simulink model "G6A_Einstiegsaufgabe_Informationstechnik1"  (R2018b)
settings: Solver=FixedStepDiscrete  StartTime=0.0  StopTime=10.0  RelTol=1e-3  EnableMultiTasking=on
libraries: commutil2 x12, c280xlib x3, c2833xlib x2, powerlib_extras x2, c2000lib x1
settings Model: ExtModeTrigDuration=8  Creator=maxth  LastModifiedBy=maxth
settings SolverCC: AutoInsertRateTranBlk=on
settings DataIOCC: LimitDataPoints=on  SaveFormat=Array  SaveOutput=off  SaveTime=off
settings OptimizationCC: DefaultUnderspecifiedDataType=single  ExpressionDepthLimit=2147483647  LifeSpan=1  MaxStackSize=512
settings DebuggingCC: UnderspecifiedInitializationDetection=Classic  MergeDetectMultiDrivingBlocksExec=none  SolverPrmCheckMsg=warning  StateNameClashWarn=warning  SFUnexpectedBacktrackingDiag=warning  SFNoUnconditionalDefaultTransitionDiag=warning  SFExecutionAtInitializationDiag=none
settings HardwareCC: ProdBitPerChar=16  ProdBitPerInt=16  ProdBitPerPointer=32  ProdBitPerSizeT=32  ProdBitPerPtrDiffT=32  ProdLargestAtomicInteger=Integer  ProdLargestAtomicFloat=None  ProdWordSize=16  ProdLongLongMode=on  ProdHWDeviceType=Texas Instruments->C2000  TargetBitPerChar=16  TargetBitPerInt=16  TargetLargestAtomicInteger=Integer  TargetIntDivRoundTo=Zero  TargetEndianess=LittleEndian  TargetWordSize=16  TargetHWDeviceType=Texas Instruments->C2000  ProdEqTarget=off
settings ModelReferenceCC: PropagateSignalLabelsOutOfModel=off
settings SFSimCC: SimCustomSourceCode="#include \"i2c_reset.c\""  SimCustomHeaderCode="#include \"i2c_reset.h\""  SimUseLocalCustomCode=off  MATLABDynamicMemAlloc=off
settings RTWCC: SystemTargetFile=ert.tlc  HardwareBoard=TI Delfino F2833x  TemplateMakefile=ert_default_tmf  RTWUseLocalCustomCode=off  RTWUseSimCustomCode=on  CustomSourceCode="#include \"i2c_reset.c\""  CustomHeaderCode="#include \"i2c_reset.h\""  Toolchain=Texas Instruments Code Composer Studio (C2000)
settings CodeAppCC: IgnoreCustomStorageClasses=off  CustomSymbolStrType=$N$R$M  StateflowObjectComments=on  InternalIdentifier=Classic
settings ERTTargetCC: CodeReplacementLibrary=TI C28x  MultiwordLength=2048  ParMdlRefBuildCompliant=off  CPPClassGenCompliant=off  ConvertIfToSwitch=off  SuppressUnreachableDefaultCases=off
settings ConfigComp: CovMetricSettings=dw  CovHtmlReporting=on  CovSaveCumulativeToWorkspaceVar=on  CovSaveSingleToWorkspaceVar=on  CovExternalEMLEnable=off

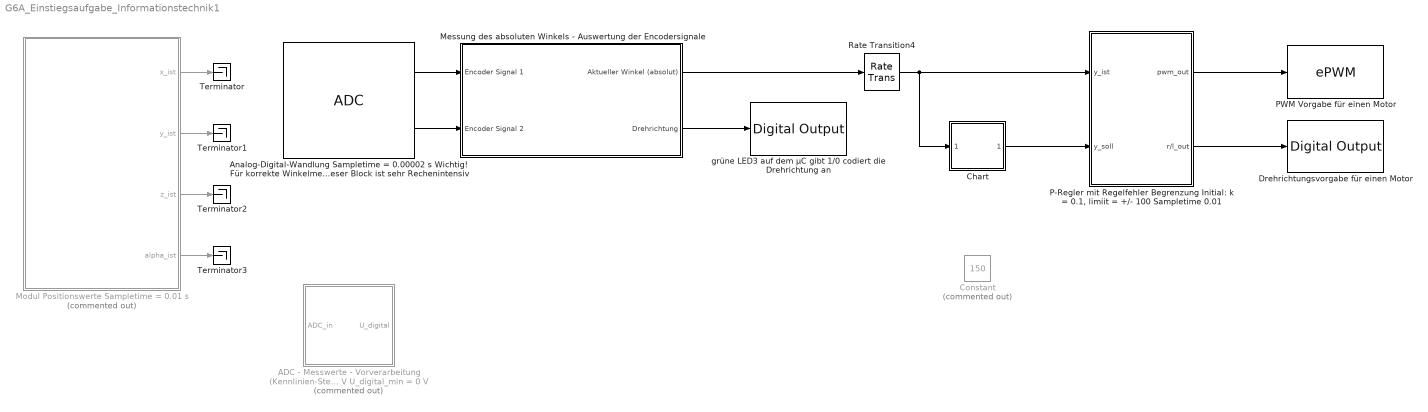
== system G6A_Einstiegsaufgabe_Informationstechnik1 ==
  ADC - Messwerte - Vorverarbeitung (Kennlinien-Steigung und Offset-Kompensation) U_digital = (ADC_in - Offset) * 3.546 V / 4096 mit U_digital_max = 3.546 V U_digital_min = 0 V : Subsystem  Commented=on
  "Analog-Digital-Wandlung Sampletime = 0.00002 s Wichtig! Für korrekte Winkelmessung nicht die Sampletime vergrößern Weitere Ports können hinzugefügt werden (Farbsensor, Sharp-Sensoren) Wichtig! Dieser Block ist sehr Rechenintensiv" : c280xlib/ADC  useModule=A  useMode=Sequential  sourceSOC=Software  sourceSOC1=Software  sourceSOC2=ePWMxB  xint2_ADCSOC=31  Ts=0.00002  dType=double  postInterrupt=off  numConversionsSingle=2  numConversionsDouble=1  conv0=ADCINA0  conv1=ADCINA1  conv2=ADCINA2  conv3=ADCINA3  conv4=ADCINA4  conv5=ADCINA5  conv6=ADCINA6  conv7=ADCINA7  conv8=ADCINB0  conv9=ADCINB1  conv10=ADCINB2  conv11=ADCINB3  conv12=ADCINB4  conv13=ADCINB5  conv14=ADCINB6  conv15=ADCINB7  convAB0=ADCINA0 and ADCINB0  convAB1=ADCINA1 and ADCINB1  convAB2=ADCINA2 and ADCINB2  convAB3=ADCINA3 and ADCINB3  convAB4=ADCINA4 and ADCINB4  convAB5=ADCINA5 and ADCINB5  convAB6=ADCINA6 and ADCINB6  convAB7=ADCINA7 and ADCINB7  convA0=ADCINA0  convA1=ADCINA1  convA2=ADCINA5  convA3=ADCINA3  convA4=ADCINA5  convA5=ADCINA5  convA6=ADCINA6  convA7=ADCINA7  convB0=ADCINB0  convB1=ADCINB1  convB2=ADCINB2  convB3=ADCINB3  convB4=ADCINB4  convB5=ADCINB5  convB6=ADCINB6  convB7=ADCINB7  c28xmultiPort=on  endma=off  chdma=1
      settings: SourceProductName=Embedded Coder Support Package for Texas Instruments C2000 Processors  SourceProductBaseCode=TIC2000
  Chart : Stateflow chart  TreatAsAtomicUnit=on
  Constant : Constant  Commented=on  Value=150
  Drehrichtungsvorgabe für einen Motor : c2833xlib/Digital Output  GPIO_Number=GPIO16~GPIO23  GPIO_Bit0=off  GPIO_BIT0_Toggle=off  GPIO_Bit1=off  GPIO_BIT1_Toggle=off  GPIO_Bit2=off  GPIO_BIT2_Toggle=off  GPIO_Bit3=off  GPIO_BIT3_Toggle=off  GPIO_Bit4=off  GPIO_BIT4_Toggle=off  GPIO_Bit5=on  GPIO_BIT5_Toggle=off  GPIO_Bit6=off  GPIO_BIT6_Toggle=off  GPIO_Bit7=off  GPIO_BIT7_Toggle=off
      settings: SourceProductName=Embedded Coder Support Package for Texas Instruments C2000 Processors  SourceProductBaseCode=TIC2000
  Messung des absoluten Winkels - Auswertung der Encodersignale : Subsystem
  Modul Positionswerte Sampletime = 0.01 s : Subsystem  Commented=on
  "P-Regler mit Regelfehler Begrenzung Initial: k = 0.1, limiit = +/- 100 Sampletime 0.01" : Subsystem
  "PWM Vorgabe für einen Motor " : c280xlib/ePWM  checkMode=off  useModule=ePWM2  periodUnits=Clock cycles  timerSource=Specify via dialog  timerPeriod_clk=64000  timerPeriod_sec=0.0001  tbshadow=Counter equals to zero  countingMode=Up  phaseActiveEnable=Disable  phaseDirection=Count down after sync  phaseActive=0  synchronizationEnable=off  synchronizationOption=Disable  clockPrescale=1  HSclockPrescale=1  ePWMxAStatus=off  CMPAUnits=Clock cycles  CMPASource=Specify via dialog  CMPAValue_per=50  CMPAValue_clk=32000  enCMPAshadow=Counter equals to zero  ePWMxAactionLogic1=Do nothing  ePWMxAactionLogic2=Clear  ePWMxAactionLogic3=Set  ePWMxAactionLogic4=Do nothing  ePWMxAactionLogic5=Do nothing  ePWMxAactionLogic6=Do nothing  ePWMxALoadMode=Load on counter equals to zero (CTR=Zero)  ePWMxACSFenable=off  ePWMxACSFvalue=Forcing disable  ePWMxASFreload=Zero  enHRPWM=off  HRPWM_LoadMode=Counter equals to zero (CTR=ZERO)  HRPWM_CTLMode=Phase control mode  HRPWM_EDGMode=Both edge  enSFO=on  ePWMxBStatus=on  CMPBUnits=Percentages  CMPBSource=Input port  CMPBValue_per=0  CMPBValue_clk=32000  enCMPBshadow=Counter equals to zero  ePWMxBactionLogic1=Do nothing  ePWMxBactionLogic2=Set  ePWMxBactionLogic3=Do nothing  ePWMxBactionLogic4=Do nothing  ePWMxBactionLogic5=Clear  ePWMxBactionLogic6=Do nothing  ePWMxBLoadMode=Load on counter equals to zero (CTR=Zero)  ePWMxBCSFenable=off  ePWMxBCSFvalue=Forcing disable  ePWMxBSFreload=Zero  enableDBePWMxA=off  enableDBePWMxB=off  DBpolarity=Active high (AH)  DBedgeDelay=Positive  DBSource_ePWMxA=ePWMxA  DBSource_ePWMxB=ePWMxA  DBperiodSource=Specify via dialog  REDperiod=0  FEDperiod=0  adcstartModuleA=off  adcrequestEventA=First event  adcstartEventA=Counter equals to zero (CTR=Zero)  adcstartModuleB=off  adcrequestEventB=First event  adcstartEventB=Counter equals to zero (CTR=Zero)  intEn=off  intPrd=First event  intSel=Counter equals to zero (CTR=Zero)  chopperEnable=off  chopperFrequency=1  chopperFirstwidth=1  chopperDuty=12.5%  tripZonesource=Specify via dialog  tzselOSHT1=off  tzselOSHT2=off  tzselOSHT3=off  tzselOSHT4=off  tzselOSHT5=off  tzselOSHT6=off  tzselCBC1=off  tzselCBC2=off  tzselCBC3=off  tzselCBC4=off  tzselCBC5=off  tzselCBC6=off  enTzOstIntr=off  enTzCbcIntr=off  ePWMxAforced=No action  ePWMxBforced=No action  timerPeriod=-1  ePWMxAValue=0  ePWMxBValue=0  tripZoneoption=One-shot trip (OSHT)
      settings: SourceProductName=Embedded Coder Support Package for Texas Instruments C2000 Processors  SourceProductBaseCode=TIC2000
  Rate Transition4 : RateTransition  OutPortSampleTime=0.01
  Terminator{,1..3} (4 alike) : Terminator
  grüne LED3 auf dem µC gibt 1/0 codiert die Drehrichtung an : c2833xlib/Digital Output  GPIO_Number=GPIO32~GPIO39  GPIO_Bit0=off  GPIO_BIT0_Toggle=off  GPIO_Bit1=off  GPIO_BIT1_Toggle=off  GPIO_Bit2=on  GPIO_BIT2_Toggle=off  GPIO_Bit3=off  GPIO_BIT3_Toggle=off  GPIO_Bit4=off  GPIO_BIT4_Toggle=off  GPIO_Bit5=off  GPIO_BIT5_Toggle=off  GPIO_Bit6=off  GPIO_BIT6_Toggle=off  GPIO_Bit7=off  GPIO_BIT7_Toggle=off
      settings: SourceProductName=Embedded Coder Support Package for Texas Instruments C2000 Processors  SourceProductBaseCode=TIC2000
  wires:
  "Analog-Digital-Wandlung Sampletime = 0.00002 s Wichtig! Für korrekte Winkelmessung nicht die Sampletime vergrößern Weitere Ports können hinzugefügt werden (Farbsensor, Sharp-Sensoren) Wichtig! Dieser Block ist sehr Rechenintensiv"/2 -> Messung des absoluten Winkels - Auswertung der Encodersignale/2(Encoder Signal 2)
  "P-Regler mit Regelfehler Begrenzung Initial: k = 0.1, limiit = +/- 100 Sampletime 0.01"/2(r/l_out) -> Drehrichtungsvorgabe für einen Motor/1
  Messung des absoluten Winkels - Auswertung der Encodersignale/1(Aktueller Winkel (absolut)) -> Rate Transition4/1
  "Analog-Digital-Wandlung Sampletime = 0.00002 s Wichtig! Für korrekte Winkelmessung nicht die Sampletime vergrößern Weitere Ports können hinzugefügt werden (Farbsensor, Sharp-Sensoren) Wichtig! Dieser Block ist sehr Rechenintensiv"/1 -> Messung des absoluten Winkels - Auswertung der Encodersignale/1(Encoder Signal 1)
  Messung des absoluten Winkels - Auswertung der Encodersignale/2(Drehrichtung) -> grüne LED3 auf dem µC gibt 1/0 codiert die Drehrichtung an/1
  "P-Regler mit Regelfehler Begrenzung Initial: k = 0.1, limiit = +/- 100 Sampletime 0.01"/1(pwm_out) -> "PWM Vorgabe für einen Motor "/1
  Modul Positionswerte Sampletime = 0.01 s/1(x_ist) -> Terminator/1
  Modul Positionswerte Sampletime = 0.01 s/2(y_ist) -> Terminator1/1
  Modul Positionswerte Sampletime = 0.01 s/3(z_ist) -> Terminator2/1
  Modul Positionswerte Sampletime = 0.01 s/4(alpha_ist) -> Terminator3/1
  Rate Transition4/1 -> Chart/1(change), "P-Regler mit Regelfehler Begrenzung Initial: k = 0.1, limiit = +/- 100 Sampletime 0.01"/1(y_ist)
  Chart/1(angle) -> "P-Regler mit Regelfehler Begrenzung Initial: k = 0.1, limiit = +/- 100 Sampletime 0.01"/2(y_soll)

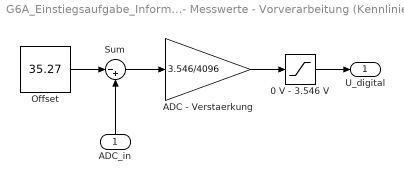
== system G6A_Einstiegsaufgabe_Informationstechnik1/ADC - Messwerte - Vorverarbeitung (Kennlinien-Steigung und Offset-Kompensation) U_digital = (ADC_in - Offset) * 3.546 V // 4096 mit U_digital_max = 3.546 V U_digital_min = 0 V ==
  ADC_in : Inport
  0 V - 3.546 V : Saturate  UpperLimit=3.546  LowerLimit=0
  ADC - Verstaerkung : Gain  Gain=3.546/4096
  Offset : Constant  Value=35.27
  Sum : Sum  Inputs=|-+
  U_digital : Outport
  wires:
  ADC - Verstaerkung/1 -> 0 V - 3.546 V/1
  Sum/1 -> ADC - Verstaerkung/1
  Offset/1 -> Sum/1
  0 V - 3.546 V/1 -> U_digital/1
  ADC_in/1 -> Sum/2

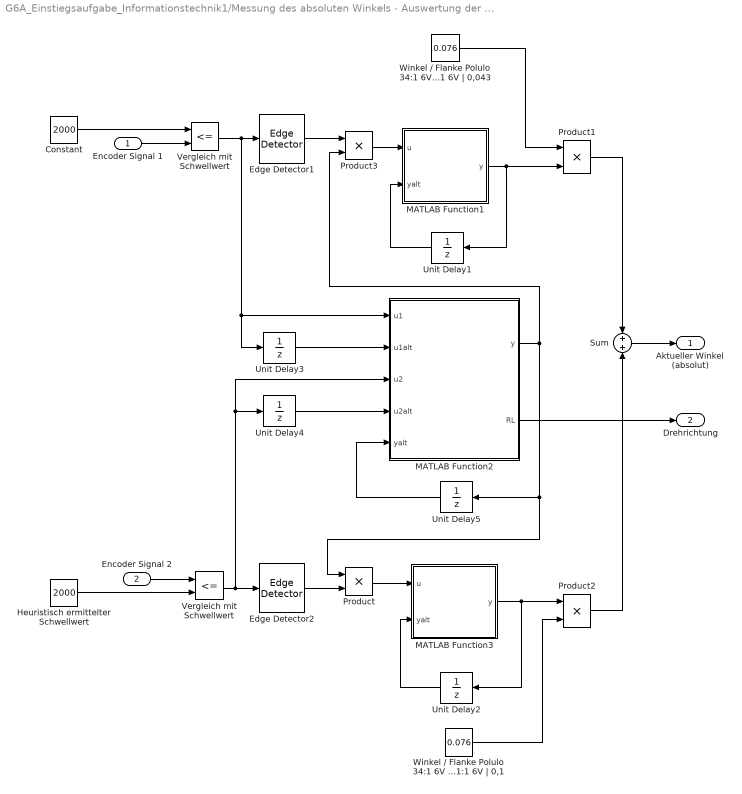
== system G6A_Einstiegsaufgabe_Informationstechnik1/Messung des absoluten Winkels - Auswertung der Encodersignale ==
  Encoder Signal 1 : Inport
  Encoder Signal 2 : Inport  Port=2
  Constant : Constant  Value=2000
  Edge Detector1 : powerlib_extras/Control  Blocks/Edge Detector  model=Either  ic=0
  Edge Detector2 : powerlib_extras/Control  Blocks/Edge Detector  model=Either  ic=0
  Heuristisch ermittelter Schwellwert : Constant  Value=2000
  MATLAB Function1 : MATLAB Function  TreatAsAtomicUnit=on
  MATLAB Function2 : MATLAB Function  TreatAsAtomicUnit=on
  MATLAB Function3 : MATLAB Function  TreatAsAtomicUnit=on
  Product{,1..3} (4 alike) : Product  RndMeth=Zero
  Sum : Sum  Inputs=+|+
  Unit Delay{1..5} (5 alike) : UnitDelay  SampleTime=-1
  Vergleich mit Schwellwert : RelationalOperator  Operator=<=  OutDataTypeStr=boolean  RndMeth=Nearest
  Vergleich mit Schwellwert : RelationalOperator  Operator=<=  OutDataTypeStr=boolean  RndMeth=Nearest
  Winkel / Flanke Polulo 34:1 6V | 0,22 Polulo 74:1 6V | 0,1 Polulo 98:1 6V | 0,076 Polulo 171:1 6V | 0,043 : Constant  Value=0.076
  Winkel / Flanke Polulo 34:1 6V | 0,22 Polulo 74:1 6V | 0,1 Polulo 98:1 6V | 0,076 Polulo 171:1 6V | 0,1 : Constant  Value=0.076
  Aktueller Winkel (absolut) : Outport
  Drehrichtung : Outport  Port=2
  wires:
  Vergleich mit Schwellwert/1 -> Unit Delay4/1, MATLAB Function2/3(u2), Edge Detector2/1
  Sum/1 -> Aktueller Winkel (absolut)/1
  Vergleich mit Schwellwert/1 -> Edge Detector1/1, Unit Delay3/1, MATLAB Function2/1(u1)
  Heuristisch ermittelter Schwellwert/1 -> Vergleich mit Schwellwert/2
  Unit Delay2/1 -> MATLAB Function3/2(yalt)
  Encoder Signal 1/1 -> Vergleich mit Schwellwert/2
  MATLAB Function3/1(y) -> Unit Delay2/1, Product2/1
  Product1/1 -> Sum/1
  Constant/1 -> Vergleich mit Schwellwert/1
  Encoder Signal 2/1 -> Vergleich mit Schwellwert/1
  Product2/1 -> Sum/2
  Unit Delay1/1 -> MATLAB Function1/2(yalt)
  MATLAB Function1/1(y) -> Product1/2, Unit Delay1/1
  Winkel / Flanke Polulo 34:1 6V | 0,22 Polulo 74:1 6V | 0,1 Polulo 98:1 6V | 0,076 Polulo 171:1 6V | 0,043/1 -> Product1/1
  Product3/1 -> MATLAB Function1/1(u)
  Product/1 -> MATLAB Function3/1(u)
  Edge Detector1/1 -> Product3/1
  Unit Delay3/1 -> MATLAB Function2/2(u1alt)
  Unit Delay4/1 -> MATLAB Function2/4(u2alt)
  Edge Detector2/1 -> Product/2
  MATLAB Function2/1(y) -> Product/1, Unit Delay5/1, Product3/2
  Winkel / Flanke Polulo 34:1 6V | 0,22 Polulo 74:1 6V | 0,1 Polulo 98:1 6V | 0,076 Polulo 171:1 6V | 0,1/1 -> Product2/2
  MATLAB Function2/2(RL) -> Drehrichtung/1
  Unit Delay5/1 -> MATLAB Function2/5(yalt)

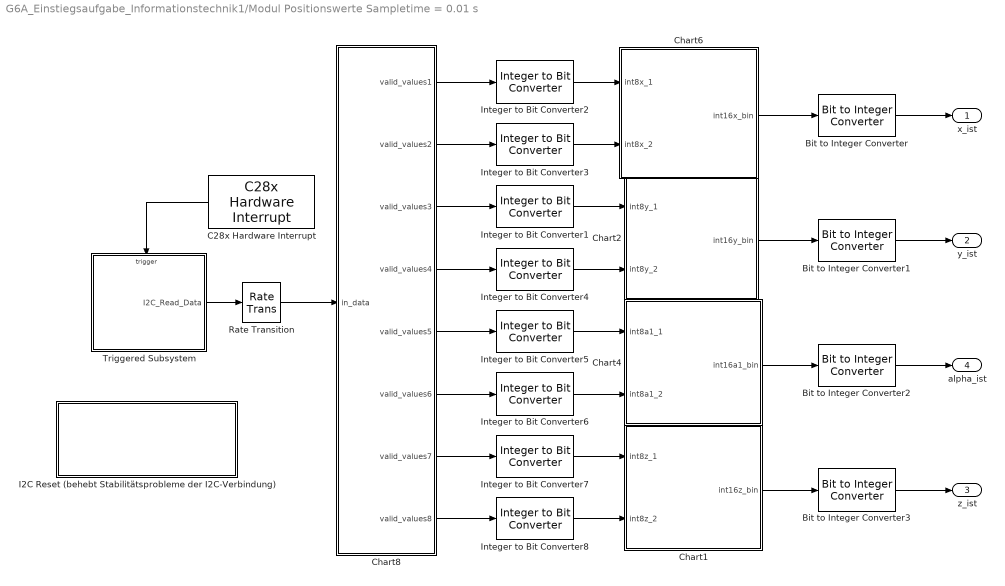
== system G6A_Einstiegsaufgabe_Informationstechnik1/Modul Positionswerte Sampletime = 0.01 s ==
  Bit to Integer Converter{,1..3} (4 alike) : commutil2/Bit to Integer Converter  nbits=16  bitOrder=MSB first  signedOutputValues=Signed  outDtype=Inherit via internal rule  outDtypeSigned=Inherit via internal rule
      settings: SourceProductName=Communications Toolbox
  C28x Hardware Interrupt : c2000lib/Scheduling/C28x Hardware Interrupt  irqnumbers=8  pienumbers=2  irqpriorities=30  irqpreempts=0  showinput=off  dspchiptype=C280X
      settings: SourceProductName=Embedded Coder Support Package for Texas Instruments C2000 Processors  SourceProductBaseCode=TIC2000
  Chart1 : Stateflow chart  TreatAsAtomicUnit=on
  Chart2 : Stateflow chart  TreatAsAtomicUnit=on
  Chart4 : Stateflow chart  TreatAsAtomicUnit=on
  Chart6 : Stateflow chart  TreatAsAtomicUnit=on
  Chart8 : Stateflow chart  TreatAsAtomicUnit=on
  I2C Reset (behebt Stabilitätsprobleme der I2C-Verbindung) : Subsystem
  Integer to Bit Converter{1..8} (8 alike) : commutil2/Integer to Bit Converter  nbits=8  signedInputValues=Unsigned  bitOrder=MSB first  outDtype=uint8
      settings: SourceProductName=Communications Toolbox
  Rate Transition : RateTransition  Deterministic=off  OutPortSampleTime=0.01
  Triggered Subsystem : Subsystem  TreatAsAtomicUnit=on
  x_ist : Outport
  y_ist : Outport  Port=2
  z_ist : Outport  Port=3
  alpha_ist : Outport  Port=4
  wires:
  Integer to Bit Converter7/1 -> Chart1/1(int8z_1)
  Integer to Bit Converter8/1 -> Chart1/2(int8z_2)
  Chart8/7(valid_values7) -> Integer to Bit Converter7/1
  Chart8/8(valid_values8) -> Integer to Bit Converter8/1
  Bit to Integer Converter3/1 -> z_ist/1
  Triggered Subsystem/1(I2C_Read_Data) -> Rate Transition/1
  Chart1/1(int16z_bin) -> Bit to Integer Converter3/1
  Chart4/1(int16a1_bin) -> Bit to Integer Converter2/1
  Chart8/6(valid_values6) -> Integer to Bit Converter6/1
  Bit to Integer Converter2/1 -> alpha_ist/1
  Bit to Integer Converter/1 -> x_ist/1
  Integer to Bit Converter6/1 -> Chart4/2(int8a1_2)
  Integer to Bit Converter5/1 -> Chart4/1(int8a1_1)
  Bit to Integer Converter1/1 -> y_ist/1
  Integer to Bit Converter4/1 -> Chart2/2(int8y_2)
  Integer to Bit Converter2/1 -> Chart6/1(int8x_1)
  Integer to Bit Converter1/1 -> Chart2/1(int8y_1)
  Chart6/1(int16x_bin) -> Bit to Integer Converter/1
  Integer to Bit Converter3/1 -> Chart6/2(int8x_2)
  Chart8/3(valid_values3) -> Integer to Bit Converter1/1
  Chart8/1(valid_values1) -> Integer to Bit Converter2/1
  Chart2/1(int16y_bin) -> Bit to Integer Converter1/1
  Chart8/4(valid_values4) -> Integer to Bit Converter4/1
  Chart8/2(valid_values2) -> Integer to Bit Converter3/1
  Chart8/5(valid_values5) -> Integer to Bit Converter5/1
  C28x Hardware Interrupt/1 -> Triggered Subsystem/Trigger
  Rate Transition/1 -> Chart8/1(in_data)

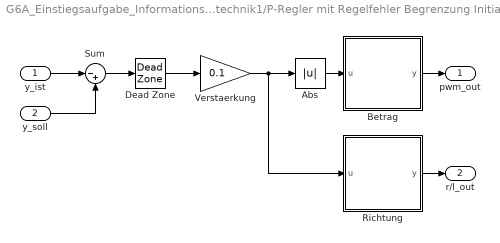
== system G6A_Einstiegsaufgabe_Informationstechnik1/P-Regler mit Regelfehler Begrenzung Initial: k = 0.1, limiit = +//- 100 Sampletime 0.01 ==
  y_ist : Inport
  y_soll : Inport  Port=2
  Abs : Abs  SampleTime=0.01
  Betrag : MATLAB Function  TreatAsAtomicUnit=on  SystemSampleTime=0.01
  Dead Zone : DeadZone  LowerValue=-100  UpperValue=100  SampleTime=0.01  SaturateOnIntegerOverflow=on
  Richtung : MATLAB Function  TreatAsAtomicUnit=on  SystemSampleTime=0.01
  Sum : Sum  Inputs=|-+  SampleTime=0.01
  Verstaerkung : Gain  Gain=0.1  SampleTime=0.01
  pwm_out : Outport
  r/l_out : Outport  Port=2
  wires:
  Betrag/1(y) -> pwm_out/1
  Verstaerkung/1 -> Abs/1, Richtung/1(u)
  Dead Zone/1 -> Verstaerkung/1
  Abs/1 -> Betrag/1(u)
  y_soll/1 -> Sum/2
  Richtung/1(y) -> r/l_out/1
  y_ist/1 -> Sum/1
  Sum/1 -> Dead Zone/1

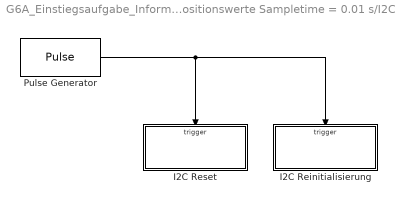
== system G6A_Einstiegsaufgabe_Informationstechnik1/Modul Positionswerte Sampletime = 0.01 s/I2C Reset (behebt Stabilitätsprobleme der I2C-Verbindung) ==
  I2C Reinitialisierung : Subsystem  TreatAsAtomicUnit=on
  I2C Reset : Subsystem  TreatAsAtomicUnit=on
  Pulse Generator : DiscretePulseGenerator  Period=250  SampleTime=0.01
  wires:
  Pulse Generator/1 -> I2C Reset/Trigger, I2C Reinitialisierung/Trigger

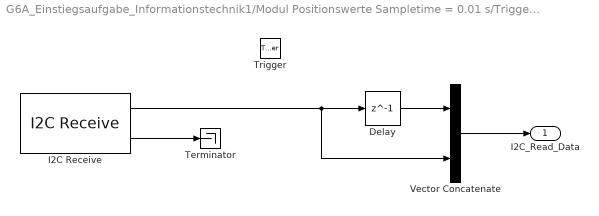
== system G6A_Einstiegsaufgabe_Informationstechnik1/Modul Positionswerte Sampletime = 0.01 s/Triggered Subsystem ==
  Trigger : TriggerPort  TriggerType=function-call  VariantControl=(inherit)
  Delay : Delay  DelayLength=1  InitialCondition=0
  I2C Receive : c280xlib/I2C Receive  selectModule=I2C_A  addrFormat=7-Bit addressing  saSource=Specify via dialog  SAR=80  bitCount=8  dataLength=10  initValue=0  NACK=on  STP=off  STR=on  sampleTime=-1  dataType=uint8
      settings: SourceProductName=Embedded Coder Support Package for Texas Instruments C2000 Processors  SourceProductBaseCode=TIC2000
  Terminator : Terminator
  Vector Concatenate : Concatenate
  I2C_Read_Data : Outport
  wires:
  I2C Receive/2 -> Terminator/1
  I2C Receive/1 -> Vector Concatenate/2, Delay/1
  Delay/1 -> Vector Concatenate/1
  Vector Concatenate/1 -> I2C_Read_Data/1

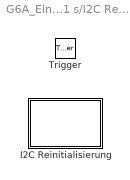
== system G6A_Einstiegsaufgabe_Informationstechnik1/Modul Positionswerte Sampletime = 0.01 s/I2C Reset (behebt Stabilitätsprobleme der I2C-Verbindung)/I2C Reinitialisierung ==
  Trigger : TriggerPort  TriggerType=falling  VariantControl=(inherit)
  I2C Reinitialisierung : MATLAB Function  TreatAsAtomicUnit=on

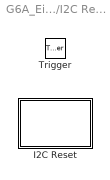
== system G6A_Einstiegsaufgabe_Informationstechnik1/Modul Positionswerte Sampletime = 0.01 s/I2C Reset (behebt Stabilitätsprobleme der I2C-Verbindung)/I2C Reset ==
  Trigger : TriggerPort  VariantControl=(inherit)
  I2C Reset : MATLAB Function  TreatAsAtomicUnit=on

== stateflow chart G6A_Einstiegsaufgabe_Informationstechnik1/Chart ==
  state Start
    angle=0;
  state Winkel1
    angle=30*2/3;
  state Winkel2
    angle=290*2/3;
  (default) -> Start
  Start -> Winkel1 : after(1,sec)
  Winkel2 -> Winkel1 : after(5,sec)[change==angle]
  Winkel1 -> Winkel2 : after(5,sec)[change==angle]
  data: angle output; change input

== matlab function G6A_Einstiegsaufgabe_Informationstechnik1/P-Regler mit Regelfehler Begrenzung Initial: k = 0.1, limiit = +//- 100 Sampletime 0.01/Betrag ==
  settings: updateMethod=DISCRETE  sampleTime=0.01
  data: u input; y output
function y = fcn( u )

if 0.5 < u && u < 60
    y = 60;
elseif u <= 0.5
    y = 0;
elseif u >= 100
    y = 100;
else
    y = abs(u);
end

== matlab function G6A_Einstiegsaufgabe_Informationstechnik1/P-Regler mit Regelfehler Begrenzung Initial: k = 0.1, limiit = +//- 100 Sampletime 0.01/Richtung ==
  settings: updateMethod=DISCRETE  sampleTime=0.01
  data: u input; y output
function y = fcn( u )

if u > 0
    y = 1;
else
    y = 0;
end

== matlab function G6A_Einstiegsaufgabe_Informationstechnik1/Messung des absoluten Winkels - Auswertung der Encodersignale/MATLAB Function1 ==
  data: u input; y output; yalt input
function y = fcn(u, yalt)

y = yalt + u;

== stateflow chart G6A_Einstiegsaufgabe_Informationstechnik1/Modul Positionswerte Sampletime = 0.01 s/Chart1 ==
  state Daten_einlesen
  state x0
  state x1_1
    entry: int16z_bin[0] = int8z_1[0];
    int16z_bin[1] = int8z_1[1];
    int16z_bin[2] = int8z_1[2];
    int16z_bin[3] = int8z_1[3];
    int16z_bin[4] = int8z_1[4];
    int16z_bin[5] = int8z_1[5]
    int16z_bin[6] = int8z_1[6];
    int16z_bin[7] = int8z_1[7];
    int16z_bin[8] = int8z_2[0];
    int16z_bin[9] = int8z_2[1];
    int16z_bin[10] = int8z_2[2];
    int16z_bin[11] = int8z_2[3];
    int16z_bin[12] = int8z_2[4];
    int16z_bin[13] = int8z_2[5]
    int16z_bin[14] = int8z_2[6];
    int16z_bin[15] = int8z_2[7];
  x0 -> Daten_einlesen
  (default) -> x0
  Daten_einlesen -> x1_1
  x1_1 -> Daten_einlesen
  data: int8z_1 input size=8; int8z_2 input size=8; int16z_bin output size=16 =0

== stateflow chart G6A_Einstiegsaufgabe_Informationstechnik1/Modul Positionswerte Sampletime = 0.01 s/Chart2 ==
  state Daten_einlesen
  state x0
  state x1_1
    entry: int16y_bin[0] = int8y_1[0];
    int16y_bin[1] = int8y_1[1];
    int16y_bin[2] = int8y_1[2];
    int16y_bin[3] = int8y_1[3];
    int16y_bin[4] = int8y_1[4];
    int16y_bin[5] = int8y_1[5]
    int16y_bin[6] = int8y_1[6];
    int16y_bin[7] = int8y_1[7];
    int16y_bin[8] = int8y_2[0];
    int16y_bin[9] = int8y_2[1];
    int16y_bin[10] = int8y_2[2];
    int16y_bin[11] = int8y_2[3];
    int16y_bin[12] = int8y_2[4];
    int16y_bin[13] = int8y_2[5]
    int16y_bin[14] = int8y_2[6];
    int16y_bin[15] = int8y_2[7];
  x0 -> Daten_einlesen
  (default) -> x0
  Daten_einlesen -> x1_1
  x1_1 -> Daten_einlesen
  data: int8y_1 input size=8; int8y_2 input size=8; int16y_bin output size=16 =0

== stateflow chart G6A_Einstiegsaufgabe_Informationstechnik1/Modul Positionswerte Sampletime = 0.01 s/Chart4 ==
  state Daten_einlesen
  state x0
  state x1_1
    entry: int16a1_bin[0] = int8a1_1[0];
    int16a1_bin[1] = int8a1_1[1];
    int16a1_bin[2] = int8a1_1[2];
    int16a1_bin[3] = int8a1_1[3];
    int16a1_bin[4] = int8a1_1[4];
    int16a1_bin[5] = int8a1_1[5]
    int16a1_bin[6] = int8a1_1[6];
    int16a1_bin[7] = int8a1_1[7];
    int16a1_bin[8] = int8a1_2[0];
    int16a1_bin[9] = int8a1_2[1];
    int16a1_bin[10] = int8a1_2[2];
    int16a1_bin[11] = int8a1_2[3];
    int16a1_bin[12] = int8a1_2[4];
    int16a1_bin[13] = int8a1_2[5]
    int16a1_bin[14] = int8a1_2[6];
    int16a1_bin[15] = int8a1_2[7];
  x0 -> Daten_einlesen
  (default) -> x0
  Daten_einlesen -> x1_1
  x1_1 -> Daten_einlesen
  data: int8a1_1 input size=8; int8a1_2 input size=8; int16a1_bin output size=16 =0

== matlab function G6A_Einstiegsaufgabe_Informationstechnik1/Messung des absoluten Winkels - Auswertung der Encodersignale/MATLAB Function2 ==
  data: u1 input; u1alt input; u2 input; u2alt input; y output; yalt input double; RL output
function [y, RL] = fcn(u1, u1alt, u2, u2alt, yalt)

y = 1;
RL = 1;

if u1alt == 0 && u2alt == 0 && u1 == 0 && u2 == 0
    y = yalt;
end

if u1alt == 0 && u2alt == 0 && u1 == 0 && u2 == 1
    y = 1;
end

if u1alt == 0 && u2alt == 0 && u1 == 1 && u2 == 0
    y = -1;
end

% if u1alt == 0 && u2alt == 0 && u1 == 1 && u2 == 1
%     y = yalt;   % nicht möglich
% end

if u1alt == 0 && u2alt == 1 && u1 == 0 && u2 == 0
    y = -1;
end

if u1alt == 0 && u2alt == 1 && u1 == 0 && u2 == 1
    y = yalt;
end

% if u1alt == 0 && u2alt == 1 && u1 == 1 && u2 == 0
%     y = yalt;   % nicht möglich
% end

if u1alt == 0 && u2alt == 1 && u1 == 1 && u2 == 1
    y = 1;
end

if u1alt == 1 && u2alt == 0 && u1 == 0 && u2 == 0
    y = 1;
end

% if u1alt == 1 && u2alt == 0 && u1 == 0 && u2 == 1
%     y = yalt;   % nicht möglich
% end

if u1alt == 1 && u2alt == 0 && u1 == 1 && u2 == 0
    y = yalt;
end

if u1alt == 1 && u2alt == 0 && u1 == 1 && u2 == 1
    y = -1;
end

% if u1alt == 1 && u2alt == 1 && u1 == 0 && u2 == 0
%     y = yalt;   % nicht möglich
% end

if u1alt == 1 && u2alt == 1 && u1 == 0 && u2 == 1
    y = -1;
end

if u1alt == 1 && u2alt == 1 && u1 == 1 && u2 == 0
    y = 1;
end

if u1alt == 1 && u2alt == 1 && u1 == 1 && u2 == 1
    y = yalt;
end

if y == 1
    RL = 1;
else
    RL = 0;
end

== stateflow chart G6A_Einstiegsaufgabe_Informationstechnik1/Modul Positionswerte Sampletime = 0.01 s/Chart6 ==
  state Daten_einlesen
  state x0
  state x1_1
    entry: int16x_bin[0] = int8x_1[0];
    int16x_bin[1] = int8x_1[1];
    int16x_bin[2] = int8x_1[2];
    int16x_bin[3] = int8x_1[3];
    int16x_bin[4] = int8x_1[4];
    int16x_bin[5] = int8x_1[5]
    int16x_bin[6] = int8x_1[6];
    int16x_bin[7] = int8x_1[7];
    int16x_bin[8] = int8x_2[0];
    int16x_bin[9] = int8x_2[1];
    int16x_bin[10] = int8x_2[2];
    int16x_bin[11] = int8x_2[3];
    int16x_bin[12] = int8x_2[4];
    int16x_bin[13] = int8x_2[5]
    int16x_bin[14] = int8x_2[6];
    int16x_bin[15] = int8x_2[7];
  x0 -> Daten_einlesen
  (default) -> x0
  Daten_einlesen -> x1_1
  x1_1 -> Daten_einlesen
  data: int8x_1 input size=8; int8x_2 input size=8; int16x_bin output size=16 =0

== stateflow chart G6A_Einstiegsaufgabe_Informationstechnik1/Modul Positionswerte Sampletime = 0.01 s/Chart8 ==
  state wert_erkannt
    entry:
    values_out1[0] = in_data[0];
    values_out1[1] = in_data[1];
    values_out1[2] = in_data[2];
    values_out1[3] = in_data[3];
    values_out1[4] = in_data[4];
    values_out1[5] = in_data[5];
    values_out1[6] = in_data[6];
    values_out1[7] = in_data[7];
    values_out1[8] = in_data[8];
    values_out1[9] = in_data[9];
    values_out1[10] = in_data[10];
    values_out1[11] = in_data[11];
    values_out1[12] = in_data[12];
    values_out1[13] = in_data[13];
    values_out1[14] = in_data[14];
    values_out1[15] = in_data[15];
    values_out1[16] = in_data[16];
    values_out1[17] = in_data[17];
    values_out1[18] = in_data[18];
    values_out1[19] = in_data[19];
  state init
    entry: values_out1[0] = 0;
    values_out1[1] = 0;
    values_out1[2] = 0;
    values_out1[3] = 0;
    values_out1[4] = 0;
    values_out1[5] = 0;
    values_out1[6] = 0;
    values_out1[7] = 0;
    values_out1[8] = 0;
    values_out1[9] = 0;
    values_out1[10] = 0;
    values_out1[11] = 0;
    values_out1[12] = 0;
    values_out1[13] = 0;
    values_out1[14] = 0;
    values_out1[15] = 0;
    values_out1[16] = 0;
    values_out1[17] = 0;
    values_out1[18] = 0;
    values_out1[19] = 0;
  state Anfang_found_Schritt_uebertragen_weglassen_performance
    entry: x_found = x_found +1;
  state x5_valid_data_found1
    entry: valid_values1 = values_out1[search+1];
    valid_values2 = values_out1[search+2];
    valid_values3 = values_out1[search+3];
    valid_values4 = values_out1[search+4];
    valid_values5 = values_out1[search+5];
    valid_values6 = values_out1[search+6];
    valid_values7 = values_out1[search+7];
    valid_values8 = values_out1[search+8];
    zaehler = zaehler +1;
  state wert_erkannt2
    entry:
    search = 0;
    counter = counter + 1;
  state x1_search1
    entry: search = search + 1;
  x5_valid_data_found1 -> wert_erkannt
  (default) -> init
  x1_search1 -> wert_erkannt [order 3]
  init -> wert_erkannt
  Anfang_found_Schritt_uebertragen_weglassen_performance -> x5_valid_data_found1 [order 1] : [((values_out1[search]+values_out1[search+1]+values_out1[search+2]+values_out1[search+3]+values_out1[search+4]+values_out1[search+5]+values_out1[search+6]+values_out1[search+7]+values_out1[search+8])) == values_out1[search+9]]
  Anfang_found_Schritt_uebertragen_weglassen_performance -> x5_valid_data_found1 [order 2] : [((values_out1[search]+values_out1[search+1]+values_out1[search+2]+values_out1[search+3]+values_out1[search+4]+values_out1[search+5]+values_out1[search+6]+values_out1[search+7]+values_out1[search+8])-(256)) == values_out1[search+9]]
  wert_erkannt -> wert_erkannt2
  Anfang_found_Schritt_uebertragen_weglassen_performance -> x5_valid_data_found1 [order 3] : [((values_out1[search]+values_out1[search+1]+values_out1[search+2]+values_out1[search+3]+values_out1[search+4]+values_out1[search+5]+values_out1[search+6]+values_out1[search+7]+values_out1[search+8])-(512)) == values_out1[search+9]]
  Anfang_found_Schritt_uebertragen_weglassen_performance -> x5_valid_data_found1 [order 7] : [((values_out1[search]+values_out1[search+1]+values_out1[search+2]+values_out1[search+3]+values_out1[search+4]+values_out1[search+5]+values_out1[search+6]+values_out1[search+7]+values_out1[search+8])-(768)) == values_out1[search+9]]
  Anfang_found_Schritt_uebertragen_weglassen_performance -> x5_valid_data_found1 [order 6] : [((values_out1[search]+values_out1[search+1]+values_out1[search+2]+values_out1[search+3]+values_out1[search+4]+values_out1[search+5]+values_out1[search+6]+values_out1[search+7]+values_out1[search+8])-(1024)) == values_out1[search+9]]
  Anfang_found_Schritt_uebertragen_weglassen_performance -> x5_valid_data_found1 [order 5] : [((values_out1[search]+values_out1[search+1]+values_out1[search+2]+values_out1[search+3]+values_out1[search+4]+values_out1[search+5]+values_out1[search+6]+values_out1[search+7]+values_out1[search+8])-(1280)) == values_out1[search+9]]
  Anfang_found_Schritt_uebertragen_weglassen_performance -> x5_valid_data_found1 [order 4] : [((values_out1[search]+values_out1[search+1]+values_out1[search+2]+values_out1[search+3]+values_out1[search+4]+values_out1[search+5]+values_out1[search+6]+values_out1[search+7]+values_out1[search+8])-(1536)) == values_out1[search+9]]
  Anfang_found_Schritt_uebertragen_weglassen_performance -> x5_valid_data_found1 [order 8] : [((values_out1[search]+values_out1[search+1]+values_out1[search+2]+values_out1[search+3]+values_out1[search+4]+values_out1[search+5]+values_out1[search+6]+values_out1[search+7]+values_out1[search+8])-(1792)) == values_out1[search+9]]
  Anfang_found_Schritt_uebertragen_weglassen_performance -> x5_valid_data_found1 [order 10] : [((values_out1[search]+values_out1[search+1]+values_out1[search+2]+values_out1[search+3]+values_out1[search+4]+values_out1[search+5]+values_out1[search+6]+values_out1[search+7]+values_out1[search+8])-(2048)) == values_out1[search+9]]
  Anfang_found_Schritt_uebertragen_weglassen_performance -> x1_search1 [order 9]
  wert_erkannt2 -> Anfang_found_Schritt_uebertragen_weglassen_performance [order 1] : [values_out1[search] == 88]
  x1_search1 -> Anfang_found_Schritt_uebertragen_weglassen_performance [order 1] : [values_out1[search] == 88]
  wert_erkannt2 -> x1_search1 [order 2]
  x1_search1 -> x1_search1 [order 2] : [search < 19]
  data: in_data input size=20; values_out1 local int16 size=20; zaehler local int32 =0; search local int16; valid_values1 output int16 size=1; valid_values2 output int16 size=1; valid_values3 output int16 size=1; valid_values4 output int16 size=1; valid_values5 output int16 size=1; valid_values6 output int16 size=1; valid_values7 output int16 size=1; valid_values8 output int16 size=1; counter local int32 =0; x_found local int32 =0

== matlab function G6A_Einstiegsaufgabe_Informationstechnik1/Messung des absoluten Winkels - Auswertung der Encodersignale/MATLAB Function3 ==
  data: u input; y output; yalt input
function y = fcn(u, yalt)

y = yalt + u;

== matlab function G6A_Einstiegsaufgabe_Informationstechnik1/Modul Positionswerte Sampletime = 0.01 s/I2C Reset (behebt Stabilitätsprobleme der I2C-Verbindung)/I2C Reset/I2C Reset ==
function fcn()
%#codegen

coder.ceval( 'reset_i2c' );

== matlab function G6A_Einstiegsaufgabe_Informationstechnik1/Modul Positionswerte Sampletime = 0.01 s/I2C Reset (behebt Stabilitätsprobleme der I2C-Verbindung)/I2C Reinitialisierung/I2C Reinitialisierung ==
function fcn()
%#codegen

coder.ceval( 'init_i2c' );
